simulink model "Model"  (R2016b)
settings: Solver=FixedStepAuto  StartTime=0.0  StopTime=10  RelTol=1e-3
values from neighbouring files (symbols this model uses):
  Ag1 = [4.1 0 0 0 0 0 0 0 0 4.3 0 0 ... (64 elements, 8x8)]    [Parameter.mat]
  Ag2 = [4.2 0 0 0 0 0 0 0 0 4.5 0 0 ... (64 elements, 8x8)]    [Parameter.mat]
  Ag3 = [5.2 0 0 0 0 0 0 0 0 5 0 0 ... (64 elements, 8x8)]    [Parameter.mat]
  Ag4 = [4.7 0 0 0 0 0 0 0 0 4.6 0 0 ... (64 elements, 8x8)]    [Parameter.mat]
  Bbl = [0 0 0 0 -0.00407136908262 0.00231264074101 -0.0023423098455 -0.00233204056557 0 0 0 0 ... (64 elements, 8x8)]    [Parameter.mat]
  Bg1 = [0.1 0.2 0.4 0.6 0 0 0 0 -0.2 -0.4 -0.8 0.7 ... (64 elements, 8x8)]    [Parameter.mat]
  Bg2 = [-0.3 0.7 0.9 0.6 0 0 0 0 0.1 -0.4 0.6 -0.5 ... (64 elements, 8x8)]    [Parameter.mat]
  Bg3 = [0.7 -1.1 -0.9 -0.1 0 0 0 0 1.2 0.3 -1.3 -0.6 ... (64 elements, 8x8)]    [Parameter.mat]
  Bg4 = [-0.5 -1.1 0.4 0.7 0 0 0 0 0.7 -0.9 0.1 -0.8 ... (64 elements, 8x8)]    [Parameter.mat]
  Cg1 = [1.1 1.2 1 -0.8 0 0 0 0 -0.6 -1.2 1 1 ... (64 elements, 8x8)]    [Parameter.mat]
  Cg2 = [0.6 -0.4 -0.3 1.2 0 0 0 0 -0.9 -1.2 -0.2 0.8 ... (64 elements, 8x8)]    [Parameter.mat]
  Cg3 = [-1.1 -0.8 1.3 -0.4 0 0 0 0 -0.3 -1.3 -0.2 -1.3 ... (64 elements, 8x8)]    [Parameter.mat]
  Cg4 = [0.8 -1.5 0.1 0.3 0 0 0 0 0.6 1.1 0.3 0.8 ... (64 elements, 8x8)]    [Parameter.mat]
  Ch1 = [0 0 0 0 0.00201847019054 -0.00145662348325 -0.00212945222702 0.00166759378573]    [Parameter.mat]
  Ch2 = [0 0 0 0 -0.00407136908262 0.00231264074101 -0.0023423098455 -0.00233204056557]    [Parameter.mat]
  Ch3 = [0 0 0 0 0.000977571145714 -0.00326431557277 0.00252790039524 -0.00249100491558]    [Parameter.mat]
  d_1 = [0 1 1 0]    [Parameter.mat]
  d_2 = [1 0 1 1]    [Parameter.mat]
  d_3 = [0 1 0 1]    [Parameter.mat]
  impulse_delay = 0.4    [Parameter.mat]
  impulse_period = 0.4    [Parameter.mat]
  L2 = [0.6 0 0 0 0 0 0 0 0 0.6 0 0 ... (64 elements, 8x8)]    [Parameter.mat]
  sampling_delay = 0.2    [Parameter.mat]
  sampling_period = 0.2    [Parameter.mat]
libraries: commrandsrc3 x3
settings Model: Creator=91542  LastModifiedBy=91542

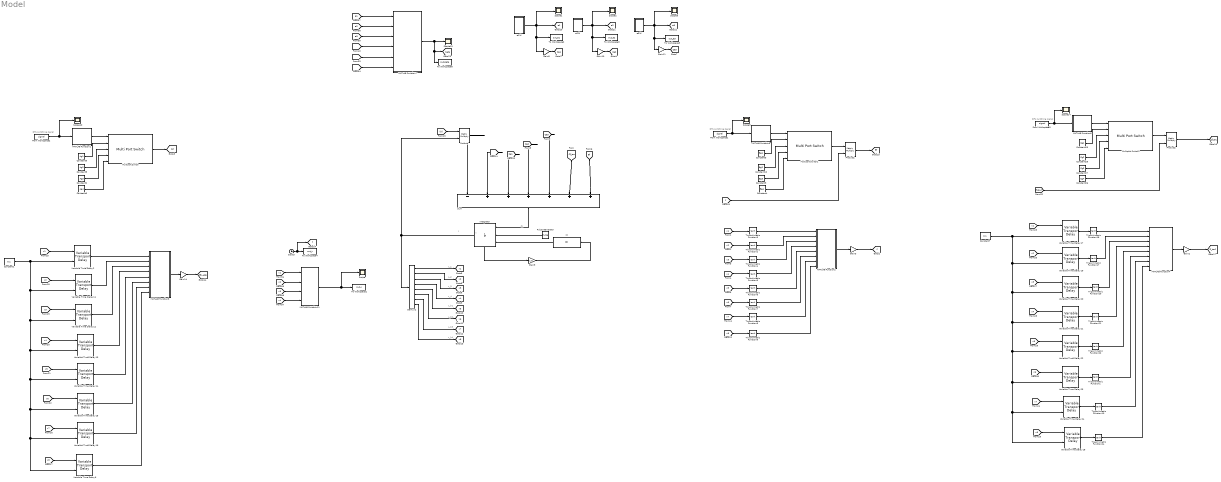
== system Model ==
  note: DFA switching signal
  note: x
  note: dx
  note: x
  note: x_1
  note: x_2
  note: x_3
  note: x_4
  note: x_h1
  note: x_h2
  note: x_h3
  note: x_h4
  note: DFA switching signal
  note: DFA switching signal
  Clock3 : Clock
  Constant1 : Constant  Value=0.1
  Constant10 : Constant  Value=Bg2
  Constant2 : Constant  Value=Ag3
  Constant25 : Constant  Value=Cg1
  Constant26 : Constant  Value=Cg4
  Constant27 : Constant  Value=Cg3
  Constant28 : Constant  Value=Cg2
  Constant3 : Constant  Value=Bg1
  Constant4 : Constant  Value=Bg4
  Constant5 : Constant  Value=Ag1
  Constant6 : Constant  Value=Ag4
  Constant7 : Constant  Value=0.1
  Constant8 : Constant  Value=Ag2
  Constant9 : Constant  Value=Bg3
  Demux2 : Demux  Outputs=8
  From Workspace1 : FromWorkspace  VariableName=signal  SampleTime=0
  From Workspace2 : FromWorkspace  VariableName=signal  SampleTime=0
  From Workspace3 : FromWorkspace  VariableName=signal  SampleTime=0
  Gain10 : Gain  Gain=Ch2  Multiplication=Matrix(K*u)
  Gain11 : Gain  Gain=Ch3  Multiplication=Matrix(K*u)
  Gain14 : Gain  Gain=Bbl  Multiplication=Matrix(K*u)
  Gain2 : Gain  Gain=L2  Multiplication=Matrix(K*u)
  Gain3 : Gain  Gain=L2  Multiplication=Matrix(K*u)
  Gain8 : Gain  Gain=Ch1  Multiplication=Matrix(K*u)
  Gain9 : Gain  Gain=1.6
  IC : InitialCondition  Value=[1.6;-1.1;1.2;-1.8;0;0;0;0];
  Integrator : Integrator  ExternalReset=rising  InitialConditionSource=external  ShowStatePort=on
  MATLAB Function1 : MATLAB Function  TreatAsAtomicUnit=on
  MATLAB Function11 : MATLAB Function  TreatAsAtomicUnit=on
  MATLAB Function2 : MATLAB Function  TreatAsAtomicUnit=on
  MATLAB Function3 : MATLAB Function  TreatAsAtomicUnit=on
  MATLAB Function4 : MATLAB Function  TreatAsAtomicUnit=on
  MATLAB Function5 : MATLAB Function  TreatAsAtomicUnit=on
  MATLAB Function6 : MATLAB Function  TreatAsAtomicUnit=on
  MATLAB Function7 : MATLAB Function  TreatAsAtomicUnit=on
  Multiport Switch : MultiPortSwitch  Inputs=4
  Multiport Switch1 : MultiPortSwitch  Inputs=4
  Multiport Switch2 : MultiPortSwitch  Inputs=4
  Product : Product  Multiplication=Matrix(*)
  Product1 : Product  Multiplication=Matrix(*)
  Product2 : Product  Multiplication=Matrix(*)
  Pulse Generator : DiscretePulseGenerator  PulseType=Time based  Amplitude=1.6  Period=impulse_period  PulseWidth=0.1  PhaseDelay=impulse_delay
  Scope{,1..3,5,10,13..14} (8 alike) : Scope
  Sum : Sum  Inputs=|-++++++
  To Workspace1 : ToWorkspace  VariableName=out_x  SaveFormat=Structure  SampleTime=-1
      settings: Save2DSignal=2-D array (concatenate along first dimension)
  To Workspace2 : ToWorkspace  VariableName=out_e1  SaveFormat=Structure  SampleTime=-1
      settings: Save2DSignal=2-D array (concatenate along first dimension)
  To Workspace3 : ToWorkspace  VariableName=out_e2  SaveFormat=Structure  SampleTime=-1
      settings: Save2DSignal=2-D array (concatenate along first dimension)
  To Workspace4 : ToWorkspace  VariableName=out_t  SaveFormat=Structure
      settings: Save2DSignal=2-D array (concatenate along first dimension)
  To Workspace5 : ToWorkspace  VariableName=out_e3  SaveFormat=Structure  SampleTime=-1
      settings: Save2DSignal=2-D array (concatenate along first dimension)
  To Workspace8 : ToWorkspace  VariableName=out_beta  SaveFormat=Structure  SampleTime=-1
      settings: Save2DSignal=2-D array (concatenate along first dimension)
  Trigonometric Function{1..10,17..18,20..22,24} (16 alike) : Trigonometry  Operator=tanh
  Variable Time Delay{2,6,11..24} (16 alike) : VariableTransportDelay  MaximumDelay=10
  e1(t) : Subsystem
  e2(t) : Subsystem
  e3(t) : Subsystem
  tag scope: Bf=global, Ce1=global, Ce2=global, Ce3=global, Cf_tau=global, beta=global, e1=global, e2=global, e3=global, f=global, t=global, x1=global, x2=global, x3=global, x4=global, x5=global, x6=global, x7=global, x8=global
  wires:
  Sum/1 -> Integrator/1
  IC/1 -> Integrator/3
  Integrator/State -> Gain9/1
  Gain9/1 -> IC/1
  [Cf_tau] -> Sum/6
  Demux2/1 -> [x1]
  Demux2/3 -> [x3]
  Demux2/4 -> [x4]
  Demux2/5 -> [x5]
  Demux2/6 -> [x6]
  Demux2/7 -> [x7]
  Demux2/8 -> [x8]
  Gain14/1 -> [Bx_eta]
  [x1] -> Variable Time Delay2/1
  [x2] -> Variable Time Delay11/1
  Variable Time Delay12/1 -> MATLAB Function3/3(F3)
  [x3] -> Variable Time Delay12/1
  Variable Time Delay13/1 -> MATLAB Function3/4(F4)
  [x4] -> Variable Time Delay13/1
  [x5] -> Variable Time Delay14/1
  [x6] -> Variable Time Delay15/1
  [x7] -> Variable Time Delay16/1
  [x8] -> Variable Time Delay6/1
  Variable Time Delay14/1 -> MATLAB Function3/5(F5)
  Variable Time Delay15/1 -> MATLAB Function3/6(F6)
  Variable Time Delay16/1 -> MATLAB Function3/7(F7)
  Variable Time Delay6/1 -> MATLAB Function3/8(F8)
  MATLAB Function3/1(y) -> Gain14/1
  MATLAB Function4/1(y) -> Gain2/1
  [x1] -> Variable Time Delay17/1
  [x2] -> Variable Time Delay19/1
  Trigonometric Function20/1 -> MATLAB Function4/3(F3)
  [x3] -> Variable Time Delay20/1
  Trigonometric Function21/1 -> MATLAB Function4/4(F4)
  [x4] -> Variable Time Delay21/1
  [x5] -> Variable Time Delay22/1
  [x6] -> Variable Time Delay23/1
  [x7] -> Variable Time Delay24/1
  [x8] -> Variable Time Delay18/1
  Trigonometric Function22/1 -> MATLAB Function4/5(F5)
  Trigonometric Function1/1 -> MATLAB Function4/6(F6)
  Trigonometric Function10/1 -> MATLAB Function4/7(F7)
  Trigonometric Function24/1 -> MATLAB Function4/8(F8)
  [x1] -> Trigonometric Function3/1
  [x2] -> Trigonometric Function2/1
  [x3] -> Trigonometric Function4/1
  [x4] -> Trigonometric Function5/1
  [x5] -> Trigonometric Function6/1
  [x6] -> Trigonometric Function7/1
  [x7] -> Trigonometric Function8/1
  [x8] -> Trigonometric Function9/1
  MATLAB Function2/1(y) -> Gain3/1
  Variable Time Delay2/1 -> MATLAB Function3/1(F1)
  Variable Time Delay11/1 -> MATLAB Function3/2(F2)
  Clock3/1 -> [t], To Workspace4/1
  Variable Time Delay17/1 -> Trigonometric Function18/1
  Variable Time Delay19/1 -> Trigonometric Function17/1
  Variable Time Delay20/1 -> Trigonometric Function20/1
  Variable Time Delay21/1 -> Trigonometric Function21/1
  Variable Time Delay22/1 -> Trigonometric Function22/1
  Variable Time Delay23/1 -> Trigonometric Function1/1
  Variable Time Delay24/1 -> Trigonometric Function10/1
  Variable Time Delay18/1 -> Trigonometric Function24/1
  [Bx_eta] -> Sum/2
  Pulse Generator/1 -> Integrator/2
  Demux2/2 -> [x2]
  From Workspace2/1 -> Scope10/1, MATLAB Function1/1(a1)
  MATLAB Function1/1(output) -> Multiport Switch/1
  Constant5/1 -> Multiport Switch/2
  Constant8/1 -> Multiport Switch/3
  Multiport Switch/1 -> [A]
  Integrator/1 -> Product/2, Demux2/1
  [A] -> Product/1
  Product/1 -> Sum/1
  From Workspace1/1 -> Scope3/1, MATLAB Function5/1(a1)
  MATLAB Function5/1(output) -> Multiport Switch1/1
  Constant3/1 -> Multiport Switch1/2
  Constant4/1 -> Multiport Switch1/5
  Constant10/1 -> Multiport Switch1/3
  Constant9/1 -> Multiport Switch1/4
  [f] -> Product1/2
  Product1/1 -> [Bf]
  Multiport Switch1/1 -> Product1/1
  From Workspace3/1 -> Scope14/1, MATLAB Function6/1(a1)
  MATLAB Function6/1(output) -> Multiport Switch2/1
  Constant25/1 -> Multiport Switch2/2
  Constant26/1 -> Multiport Switch2/5
  Constant28/1 -> Multiport Switch2/3
  Constant27/1 -> Multiport Switch2/4
  [f_tau] -> Product2/2
  Product2/1 -> [Cf_tau]
  Multiport Switch2/1 -> Product2/1
  Constant6/1 -> Multiport Switch/5
  Constant2/1 -> Multiport Switch/4
  Trigonometric Function3/1 -> MATLAB Function2/1(F1)
  Trigonometric Function2/1 -> MATLAB Function2/2(F2)
  Trigonometric Function4/1 -> MATLAB Function2/3(F3)
  Trigonometric Function5/1 -> MATLAB Function2/4(F4)
  Trigonometric Function6/1 -> MATLAB Function2/5(F5)
  Trigonometric Function7/1 -> MATLAB Function2/6(F6)
  Trigonometric Function8/1 -> MATLAB Function2/7(F7)
  Trigonometric Function9/1 -> MATLAB Function2/8(F8)
  Constant7/1 -> Variable Time Delay19/2, Variable Time Delay20/2, Variable Time Delay18/2, Variable Time Delay24/2, Variable Time Delay23/2, Variable Time Delay22/2, Variable Time Delay21/2, Variable Time Delay17/2
  Trigonometric Function18/1 -> MATLAB Function4/1(F1)
  Trigonometric Function17/1 -> MATLAB Function4/2(F2)
  [Ce1] -> Sum/3
  [Ce2] -> Sum/4
  [Ce3] -> Sum/5
  [Bf] -> Sum/7
  Gain3/1 -> [f]
  Gain2/1 -> [f_tau]
  Constant1/1 -> Variable Time Delay6/2, Variable Time Delay16/2, Variable Time Delay15/2, Variable Time Delay14/2, Variable Time Delay13/2, Variable Time Delay12/2, Variable Time Delay11/2, Variable Time Delay2/2
  Gain8/1 -> [Ce1]
  e1(t)/1(Out1) -> Scope1/1, [e1], Gain8/1, To Workspace2/1  "e1(t)"
  Gain10/1 -> [Ce2]
  e2(t)/1(Out2) -> Scope2/1, [e2], Gain10/1, To Workspace3/1  "e2(t)"
  e3(t)/1(Out3) -> Scope5/1, [e3], Gain11/1, To Workspace5/1  "e3(t)"
  Gain11/1 -> [Ce3]
  [x3] -> MATLAB Function11/3(F3)
  [x4] -> MATLAB Function11/4(F4)
  [x2] -> MATLAB Function11/2(F2)
  MATLAB Function11/1(y) -> Scope/1, To Workspace1/1
  [x1] -> MATLAB Function11/1(F1)
  [e1] -> MATLAB Function7/1(e1)
  [e2] -> MATLAB Function7/2(e2)
  [e3] -> MATLAB Function7/3(e3)
  MATLAB Function7/1(beta) -> To Workspace8/1, [beta], Scope13/1
  [sigma1] -> MATLAB Function7/4(sigma1)
  [sigma2] -> MATLAB Function7/5(sigma2)
  [sigma3] -> MATLAB Function7/6(sigma3)

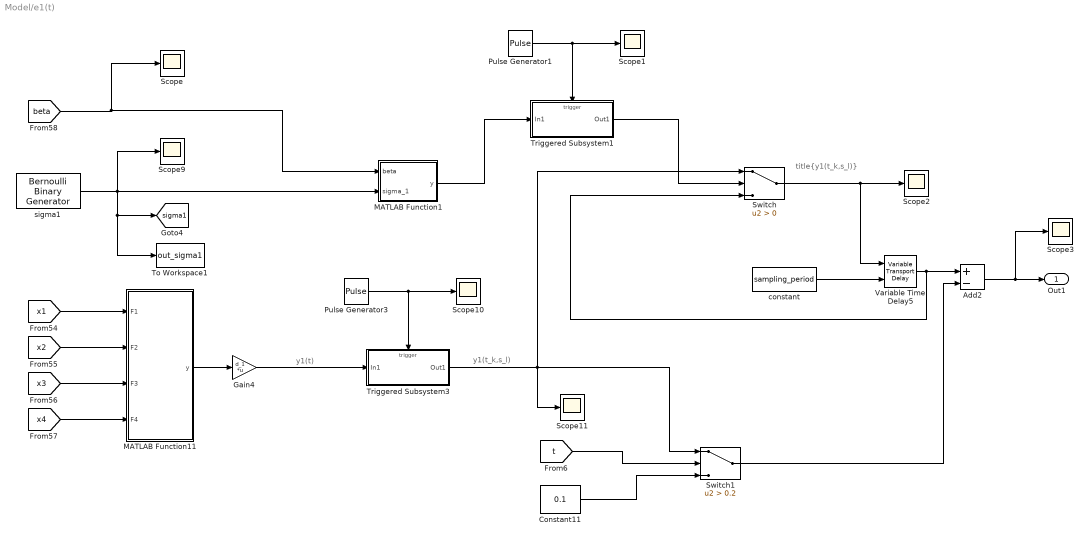
== system Model/e1(t) ==
  note: title{y1(t_k,s_l)}
  note: y1(t_k,s_l)
  note: y1(t)
  Add2 : Sum  Inputs=+-
  Constant11 : Constant  Value=0.1
  Gain4 : Gain  Gain=d_1  Multiplication=Matrix(K*u)
  MATLAB Function1 : MATLAB Function  TreatAsAtomicUnit=on
  MATLAB Function11 : MATLAB Function  TreatAsAtomicUnit=on
  Pulse Generator1 : DiscretePulseGenerator  PulseType=Time based  Period=sampling_period  PulseWidth=0.1  PhaseDelay=sampling_delay
  Pulse Generator3 : DiscretePulseGenerator  PulseType=Time based  Period=sampling_period  PulseWidth=0.1  PhaseDelay=sampling_delay
  Scope{,1..3,9..11} (7 alike) : Scope
  Switch : Switch  Criteria=u2 > Threshold
  Switch1 : Switch  Criteria=u2 > Threshold  Threshold=0.2
  To Workspace1 : ToWorkspace  VariableName=out_sigma1  SaveFormat=Structure
      settings: Save2DSignal=2-D array (concatenate along first dimension)
  Triggered Subsystem1 : Subsystem  TreatAsAtomicUnit=on
  Triggered Subsystem3 : Subsystem  TreatAsAtomicUnit=on
  Variable Time Delay5 : VariableTransportDelay  MaximumDelay=10
  constant : Constant  Value=sampling_period
  sigma1 : commrandsrc3/Bernoulli Binary Generator  ProbabilityOfZero=0.4  SeedSource=Parameter  Seed=0.5  SampleTime=0.2  SamplesPerFrame=1  OutputDataType=double  SimulateUsing=Interpreted execution
  Out1 : Outport
  tag scope: sigma1=global
  wires:
  [x3] -> MATLAB Function11/3(F3)
  Switch/1 -> Scope2/1, Variable Time Delay5/1
  constant/1 -> Variable Time Delay5/2
  Variable Time Delay5/1 -> Switch/3, Add2/1
  Triggered Subsystem3/1(Out1) -> Scope11/1, Switch1/1, Switch/1
  Switch1/1 -> Add2/2
  Constant11/1 -> Switch1/3
  Add2/1 -> Scope3/1, Out1/1
  [t] -> Switch1/2
  [x4] -> MATLAB Function11/4(F4)
  Pulse Generator3/1 -> Scope10/1, Triggered Subsystem3/Trigger
  Gain4/1 -> Triggered Subsystem3/1(In1)
  [x2] -> MATLAB Function11/2(F2)
  MATLAB Function11/1(y) -> Gain4/1
  [x1] -> MATLAB Function11/1(F1)
  [beta] -> Scope/1, MATLAB Function1/1(beta)
  sigma1/1 -> To Workspace1/1, [sigma1], MATLAB Function1/2(sigma_1), Scope9/1
  Pulse Generator1/1 -> Scope1/1, Triggered Subsystem1/Trigger
  Triggered Subsystem1/1(Out1) -> Switch/2
  MATLAB Function1/1(y) -> Triggered Subsystem1/1(In1)

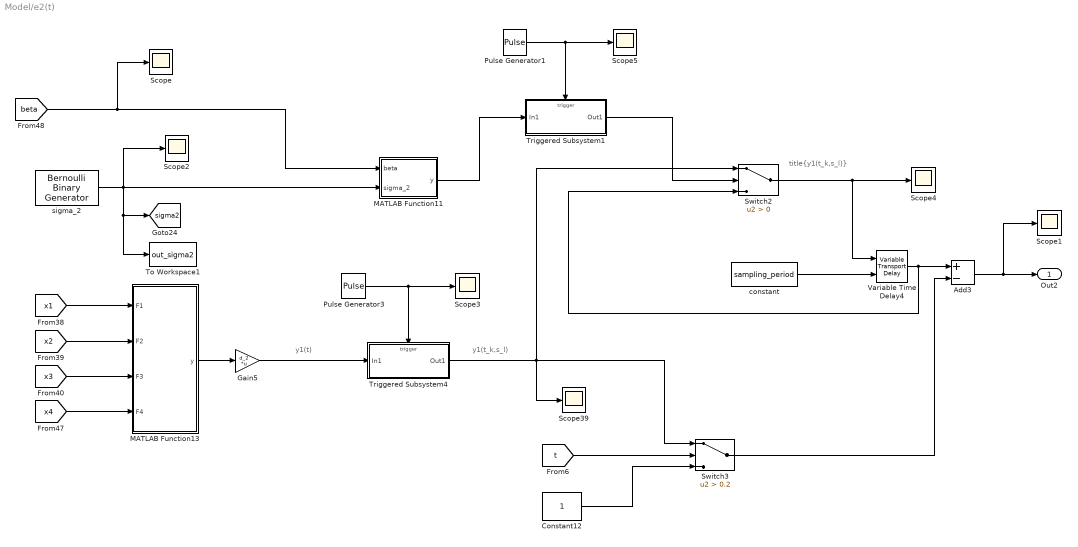
== system Model/e2(t) ==
  note: title{y1(t_k,s_l)}
  note: y1(t_k,s_l)
  note: y1(t)
  Add3 : Sum  Inputs=+-
  Constant12 : Constant
  Gain5 : Gain  Gain=d_2  Multiplication=Matrix(K*u)
  MATLAB Function11 : MATLAB Function  TreatAsAtomicUnit=on
  MATLAB Function13 : MATLAB Function  TreatAsAtomicUnit=on
  Pulse Generator1 : DiscretePulseGenerator  PulseType=Time based  Period=sampling_period  PulseWidth=0.1  PhaseDelay=sampling_delay
  Pulse Generator3 : DiscretePulseGenerator  PulseType=Time based  Period=sampling_period  PulseWidth=0.1  PhaseDelay=sampling_delay
  Scope{,1..5,39} (7 alike) : Scope
  Switch2 : Switch  Criteria=u2 > Threshold
  Switch3 : Switch  Criteria=u2 > Threshold  Threshold=0.2
  To Workspace1 : ToWorkspace  VariableName=out_sigma2  SaveFormat=Structure
      settings: Save2DSignal=2-D array (concatenate along first dimension)
  Triggered Subsystem1 : Subsystem  TreatAsAtomicUnit=on
  Triggered Subsystem4 : Subsystem  TreatAsAtomicUnit=on
  Variable Time Delay4 : VariableTransportDelay  MaximumDelay=10
  constant : Constant  Value=sampling_period
  sigma_2 : commrandsrc3/Bernoulli Binary Generator  ProbabilityOfZero=0.4  SeedSource=Parameter  Seed=1  SampleTime=0.1  SamplesPerFrame=1  OutputDataType=double  SimulateUsing=Interpreted execution
  Out2 : Outport
  tag scope: sigma2=global
  wires:
  Variable Time Delay4/1 -> Switch2/3, Add3/1
  [x1] -> MATLAB Function13/1(F1)
  Gain5/1 -> Triggered Subsystem4/1(In1)
  [beta] -> Scope/1, MATLAB Function11/1(beta)
  [x2] -> MATLAB Function13/2(F2)
  MATLAB Function13/1(y) -> Gain5/1
  [x4] -> MATLAB Function13/4(F4)
  [x3] -> MATLAB Function13/3(F3)
  Pulse Generator3/1 -> Scope3/1, Triggered Subsystem4/Trigger
  Constant12/1 -> Switch3/3
  [t] -> Switch3/2
  constant/1 -> Variable Time Delay4/2
  Switch3/1 -> Add3/2
  Switch2/1 -> Scope4/1, Variable Time Delay4/1
  Triggered Subsystem4/1(Out1) -> Switch3/1, Scope39/1, Switch2/1
  Add3/1 -> Scope1/1, Out2/1
  sigma_2/1 -> To Workspace1/1, [sigma2], MATLAB Function11/2(sigma_2), Scope2/1
  Pulse Generator1/1 -> Scope5/1, Triggered Subsystem1/Trigger
  Triggered Subsystem1/1(Out1) -> Switch2/2
  MATLAB Function11/1(y) -> Triggered Subsystem1/1(In1)

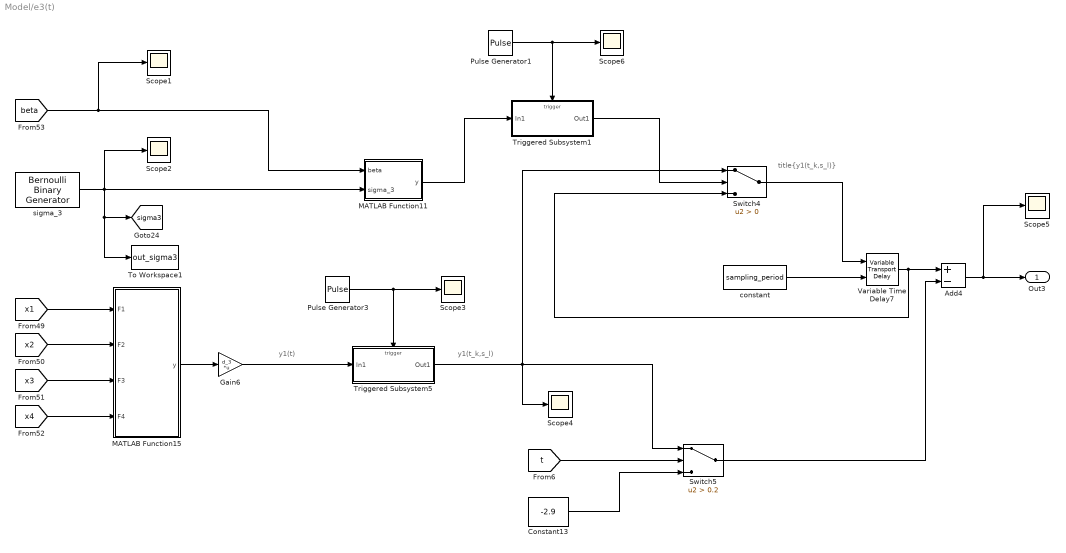
== system Model/e3(t) ==
  note: title{y1(t_k,s_l)}
  note: y1(t_k,s_l)
  note: y1(t)
  Add4 : Sum  Inputs=+-
  Constant13 : Constant  Value=-2.9
  Gain6 : Gain  Gain=d_3  Multiplication=Matrix(K*u)
  MATLAB Function11 : MATLAB Function  TreatAsAtomicUnit=on
  MATLAB Function15 : MATLAB Function  TreatAsAtomicUnit=on
  Pulse Generator1 : DiscretePulseGenerator  PulseType=Time based  Period=sampling_period  PulseWidth=0.1  PhaseDelay=sampling_delay
  Pulse Generator3 : DiscretePulseGenerator  PulseType=Time based  Period=sampling_period  PulseWidth=0.1  PhaseDelay=sampling_delay
  Scope{1..6} (6 alike) : Scope
  Switch4 : Switch  Criteria=u2 > Threshold
  Switch5 : Switch  Criteria=u2 > Threshold  Threshold=0.2
  To Workspace1 : ToWorkspace  VariableName=out_sigma3  SaveFormat=Structure
      settings: Save2DSignal=2-D array (concatenate along first dimension)
  Triggered Subsystem1 : Subsystem  TreatAsAtomicUnit=on
  Triggered Subsystem5 : Subsystem  TreatAsAtomicUnit=on
  Variable Time Delay7 : VariableTransportDelay  MaximumDelay=10
  constant : Constant  Value=sampling_period
  sigma_3 : commrandsrc3/Bernoulli Binary Generator  ProbabilityOfZero=0.6  SeedSource=Parameter  Seed=0.5  SampleTime=0.1  SamplesPerFrame=1  OutputDataType=double  SimulateUsing=Interpreted execution
  Out3 : Outport
  tag scope: sigma3=global
  wires:
  [x1] -> MATLAB Function15/1(F1)
  [x2] -> MATLAB Function15/2(F2)
  Switch5/1 -> Add4/2
  constant/1 -> Variable Time Delay7/2
  Pulse Generator3/1 -> Scope3/1, Triggered Subsystem5/Trigger
  [x3] -> MATLAB Function15/3(F3)
  [beta] -> Scope1/1, MATLAB Function11/1(beta)
  Variable Time Delay7/1 -> Switch4/3, Add4/1
  MATLAB Function15/1(y) -> Gain6/1
  [t] -> Switch5/2
  Constant13/1 -> Switch5/3
  Add4/1 -> Scope5/1, Out3/1
  [x4] -> MATLAB Function15/4(F4)
  Switch4/1 -> Variable Time Delay7/1
  Triggered Subsystem5/1(Out1) -> Scope4/1, Switch5/1, Switch4/1
  Gain6/1 -> Triggered Subsystem5/1(In1)
  sigma_3/1 -> Scope2/1, To Workspace1/1, [sigma3], MATLAB Function11/2(sigma_3)
  Pulse Generator1/1 -> Scope6/1, Triggered Subsystem1/Trigger
  Triggered Subsystem1/1(Out1) -> Switch4/2
  MATLAB Function11/1(y) -> Triggered Subsystem1/1(In1)

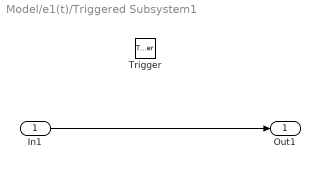
== system Model/e1(t)/Triggered Subsystem1 ==
  In1 : Inport
  Trigger : TriggerPort  VariantControl=(inherit)
  Out1 : Outport
  wires:
  In1/1 -> Out1/1

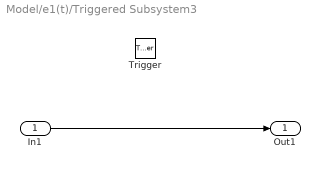
== system Model/e1(t)/Triggered Subsystem3 ==
  In1 : Inport
  Trigger : TriggerPort  VariantControl=(inherit)
  Out1 : Outport
  wires:
  In1/1 -> Out1/1

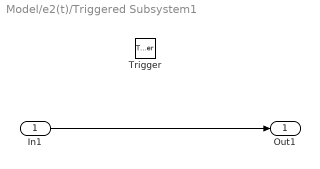
== system Model/e2(t)/Triggered Subsystem1 ==
  In1 : Inport
  Trigger : TriggerPort  VariantControl=(inherit)
  Out1 : Outport
  wires:
  In1/1 -> Out1/1

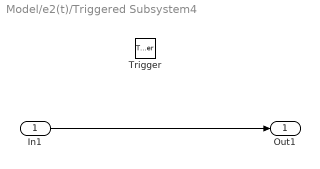
== system Model/e2(t)/Triggered Subsystem4 ==
  In1 : Inport
  Trigger : TriggerPort  VariantControl=(inherit)
  Out1 : Outport
  wires:
  In1/1 -> Out1/1

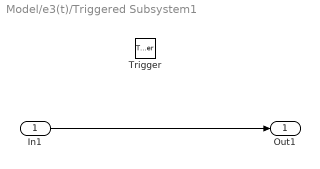
== system Model/e3(t)/Triggered Subsystem1 ==
  In1 : Inport
  Trigger : TriggerPort  VariantControl=(inherit)
  Out1 : Outport
  wires:
  In1/1 -> Out1/1

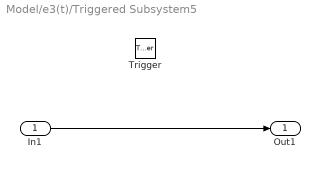
== system Model/e3(t)/Triggered Subsystem5 ==
  In1 : Inport
  Trigger : TriggerPort  VariantControl=(inherit)
  Out1 : Outport
  wires:
  In1/1 -> Out1/1

== matlab function Model/MATLAB Function11 ==
  data: F1 input; y output; F2 input; F3 input; F4 input
function y = fcn(F1,F2,F3,F4)
y =[F1;F2;F3;F4];

== matlab function Model/MATLAB Function2 ==
  data: F1 input; y output; F2 input; F3 input; F4 input; F5 input; F6 input; F7 input; F8 input
function y = fcn(F1,F2,F3,F4,F5,F6,F7,F8)
y =[F1;F2;F3;F4;F5;F6;F7;F8];

== matlab function Model/MATLAB Function7 ==
  data: e1 input; e2 input; e3 input; sigma1 input; sigma2 input; sigma3 input; beta output
function beta  = compute_beta(e1, e2, e3, sigma1, sigma2, sigma3)
    % Define initial values
    R1_init = 1080.2227;
    R2_init = 1080.2131;
    R3_init = 1080.1865; 
    
    % The feedback signals
    FB1 = 1 - sigma1;
    FB2 = 1 - sigma2;
    FB3 = 1 - sigma3;
    
    % Step 1: Calculate e_i^T * R_i * e_i
    eRi1 = e1' * R1_init * e1;
    eRi2 = e2' * R2_init * e2;
    eRi3 = e3' * R3_init * e3;
    
    % Step 2: Find the minimum value of the secure channel and the maximum value of the attacked channel
    min_val = Inf;
    max_val = -Inf;
    
    % For channel labeled 1
    if FB1 == 1 && sigma1 == 0 
        min_val = min(min_val, eRi1);
    else
        max_val = max(max_val, eRi1);
    end
    
    % For channel labeled 2
    if FB2 == 1 && sigma2 == 0
        min_val = min(min_val, eRi2);
    else
        max_val = max(max_val, eRi2);
    end
    
    % For channel labeled 3
    if FB3 == 1 && sigma3 == 0
        min_val = min(min_val, eRi3);
    else
        max_val = max(max_val, eRi3);
    end

    % Step 3: Compare the minimum and maximum values and calculate M_min
    if min_val > max_val
        M_min = 0;
    else
        M_min = max_val - min_val;
    end

    % Step 4: Update the weighting matrices
    % For R_1
    if FB1 == 1 && sigma1 == 0
        R1_new = R1_init + M_min * eye(size(R1_init));  
    else
        R1_new = R1_init;  
    end

    % For R_2
    if FB2 == 1 && sigma2 == 0
        R2_new = R2_init + M_min * eye(size(R2_init));  
    else
        R2_new = R2_init;  
    end

    % For R_3
    if FB3 == 1 && sigma3 == 0
        R3_new = R3_init + M_min * eye(size(R3_init));  
    else
        R3_new = R3_init;  
    end

    % Recalculate e_ν^T * R_ν_new * e_ν for ν = 1, 2, 3
    eR1_new = e1' * R1_new * e1;
    eR2_new = e2' * R2_new * e2;
    eR3_new = e3' * R3_new * e3;
    
    % Store all updated e_ν^T * R_ν * e_ν values in an array
    eR_vals_new = [eR1_new, eR2_new, eR3_new];

    % Take the argmax over ν = 1, 2, 3
    max_val = max(eR_vals_new);  % Find the maximum value
    candidates = find(eR_vals_new == max_val);  % Find all ν where the value equals max
    
    % Select the smallest ν among the candidates
    beta = min(candidates);  % Take the smallest index
end

== matlab function Model/MATLAB Function3 ==
  data: F1 input; y output; F2 input; F3 input; F4 input; F5 input; F6 input; F7 input; F8 input
function y = fcn(F1,F2,F3,F4,F5,F6,F7,F8)
y =[F1;F2;F3;F4;F5;F6;F7;F8];

== matlab function Model/MATLAB Function4 ==
  data: F1 input; y output; F2 input; F3 input; F4 input; F5 input; F6 input; F7 input; F8 input
function y = fcn(F1,F2,F3,F4,F5,F6,F7,F8)
y =[F1;F2;F3;F4;F5;F6;F7;F8];

== matlab function Model/MATLAB Function6 ==
  data: a1 input; output output
function output = fcn(a1)
    if (a1 == 1)
        output = 1; 
    elseif (a1 == 2)
        output = 2;
    elseif (a1 == 3)
        output = 3;
    elseif (a1 == 4)
        output = 4; 
    else
        output = 4;
    end
end

== matlab function Model/MATLAB Function1 ==
  data: a1 input; output output
function output = fcn(a1)
    if (a1 == 1)
        output = 1;
    elseif (a1 == 2)
        output = 2;
    elseif (a1 == 3)
        output = 3;
    elseif (a1 == 4)
        output = 4; 
    else
        output = 4; 
    end
end

== matlab function Model/MATLAB Function5 ==
  data: a1 input; output output
function output = fcn(a1)
    if (a1 == 1)
        output = 1; 
    elseif (a1 == 2)
        output = 2;
    elseif (a1 == 3)
        output = 3;
    elseif (a1 == 4)
        output = 4; 
    else
        output = 4; 
    end
end

== matlab function Model/e1(t)/MATLAB Function11 ==
  data: F1 input; y output; F2 input; F3 input; F4 input
function y = fcn(F1,F2,F3,F4)
y =[F1;F2;F3;F4];

== matlab function Model/e2(t)/MATLAB Function11 ==
  data: beta input; y output; sigma_2 input
function y= fcn(beta,sigma_2)
if (beta==2&&sigma_2==0)
    y=1;
else
    y=0;
end

== matlab function Model/e2(t)/MATLAB Function13 ==
  data: F1 input; y output; F2 input; F3 input; F4 input
function y = fcn(F1,F2,F3,F4)
y =[F1;F2;F3;F4];

== matlab function Model/e3(t)/MATLAB Function11 ==
  data: beta input; y output; sigma_3 input
function y= fcn(beta,sigma_3)
if (beta==3&&sigma_3==0)
    y=1;
else
    y=0;
end

== matlab function Model/e3(t)/MATLAB Function15 ==
  data: F1 input; y output; F2 input; F3 input; F4 input
function y = fcn(F1,F2,F3,F4)
y =[F1;F2;F3;F4];

== matlab function Model/e1(t)/MATLAB Function1 ==
  data: beta input; y output; sigma_1 input
function y= fcn(beta,sigma_1)
if (beta==1&&sigma_1==0)
    y=1;
else
    y=0;
end
